simulink model "PX4OutputMappingOctarotor"  (R2026a)
settings: Solver=ode4  FixedStep=stepSize_s
undefined symbols (not defined in the file): MotorCommandHexBus
settings Model: Creator=Edison Altamirano  LastModifiedBy=Edison Altamirano

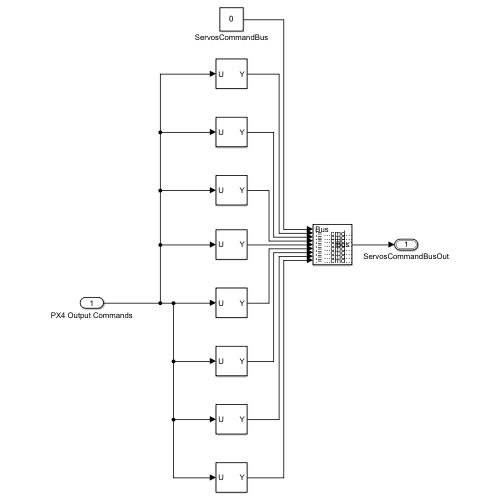
[thumbnail: Simulink's stored preview of the top-level diagram]
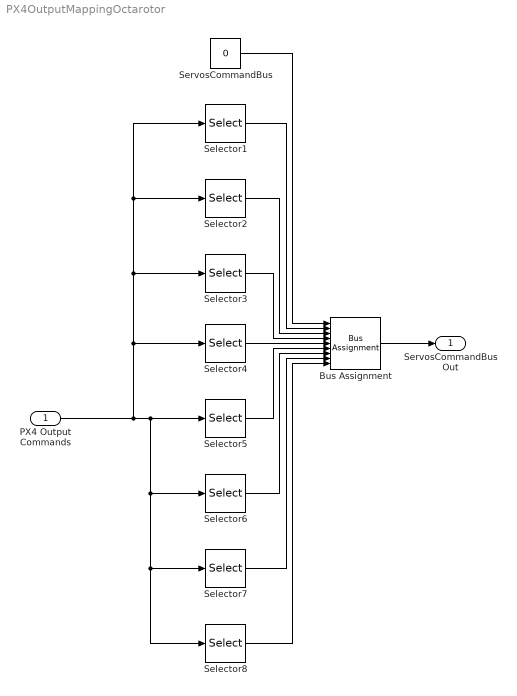
== system PX4OutputMappingOctarotor ==
  PX4 Output Commands : Inport  PortDimensions=16
  Bus Assignment : BusAssignment  AssignedSignals=MotorCommandHexBus.cmdRotor1_nd,MotorCommandHexBus.cmdRotor2_nd,MotorCommandHexBus.cmdRotor3_nd,MotorCommandHexBus.cmdRotor4_nd,MotorCommandHexBus.cmdRotor5_nd,MotorCommandHexBus.cmdRotor6_nd,MotorCommandHexBus.cmdRotor7_nd,MotorCommandHexBus.cmdRotor8_nd
  Selector1 : Selector  InputPortWidth=16  IndexOptions=Index vector (dialog)  Indices=1  OutputSizes=1
  Selector2 : Selector  InputPortWidth=16  IndexOptions=Index vector (dialog)  Indices=2  OutputSizes=1
  Selector3 : Selector  InputPortWidth=16  IndexOptions=Index vector (dialog)  Indices=3  OutputSizes=1
  Selector4 : Selector  InputPortWidth=16  IndexOptions=Index vector (dialog)  Indices=4  OutputSizes=1
  Selector5 : Selector  InputPortWidth=16  IndexOptions=Index vector (dialog)  Indices=5  OutputSizes=1
  Selector6 : Selector  InputPortWidth=16  IndexOptions=Index vector (dialog)  Indices=6  OutputSizes=1
  Selector7 : Selector  InputPortWidth=16  IndexOptions=Index vector (dialog)  Indices=7  OutputSizes=1
  Selector8 : Selector  InputPortWidth=16  IndexOptions=Index vector (dialog)  Indices=8  OutputSizes=1
  ServosCommandBus : Constant  Value=0  OutDataTypeStr=Bus: ServosCommandBus
  ServosCommandBusOut : Outport  OutDataTypeStr=Bus: ServosCommandBus
  wires:
  Bus Assignment/1 -> ServosCommandBusOut/1
  Selector8/1 -> Bus Assignment/9
  Selector7/1 -> Bus Assignment/8
  Selector6/1 -> Bus Assignment/7
  Selector5/1 -> Bus Assignment/6
  Selector4/1 -> Bus Assignment/5
  Selector3/1 -> Bus Assignment/4
  Selector2/1 -> Bus Assignment/3
  Selector1/1 -> Bus Assignment/2
  ServosCommandBus/1 -> Bus Assignment/1
  PX4 Output Commands/1 -> Selector7/1, Selector8/1, Selector6/1, Selector5/1, Selector1/1, Selector2/1, Selector3/1, Selector4/1
